simulink model "dus"  (R2014a)
settings: Solver=FixedStepDiscrete  StartTime=0.0  StopTime=10.0  FixedStep=0.1  RelTol=1e-3
settings Model: Creator=yoshi12  LastModifiedBy=yoshi12

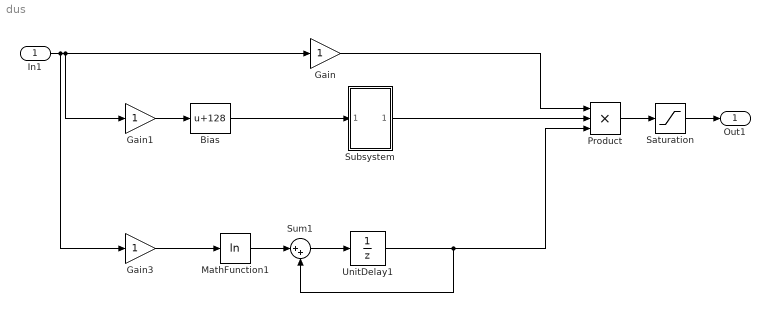
== system dus ==
  In1 : Inport
  Bias : Bias  Bias=128
  Gain : Gain
  Gain1 : Gain
  Gain3 : Gain
  MathFunction1 : Math  Operator=log  SaturateOnIntegerOverflow=on
  Product : Product  Inputs=3
  Saturation : Saturate
  Subsystem : Subsystem
  Sum1 : Sum  Inputs=|++
  UnitDelay1 : UnitDelay  SampleTime=-1
  Out1 : Outport
  wires:
  In1/1 -> Gain3/1, Gain1/1, Gain/1
  Gain/1 -> Product/1
  Product/1 -> Saturation/1
  Saturation/1 -> Out1/1
  Gain1/1 -> Bias/1
  Gain3/1 -> MathFunction1/1
  MathFunction1/1 -> Sum1/1
  UnitDelay1/1 -> Sum1/2, Product/3
  Sum1/1 -> UnitDelay1/1
  Bias/1 -> Subsystem/1(In1)
  Subsystem/1(Out1) -> Product/2

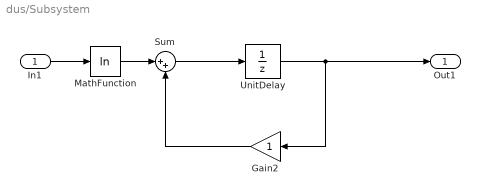
== system dus/Subsystem ==
  In1 : Inport
  Gain2 : Gain
  MathFunction : Math  Operator=log  SaturateOnIntegerOverflow=on
  Sum : Sum  Inputs=|++
  UnitDelay : UnitDelay  SampleTime=-1
  Out1 : Outport
  wires:
  Sum/1 -> UnitDelay/1
  UnitDelay/1 -> Out1/1, Gain2/1
  In1/1 -> MathFunction/1
  Gain2/1 -> Sum/2
  MathFunction/1 -> Sum/1
